simulink model "global_model"  (R2021a)
settings: Solver=ode8  StartTime=0.0  StopTime=205  FixedStep=0.1  RelTol=1e-3  EnableMultiTasking=on
undefined symbols (not defined in the file or in its folder): sigbuilder_block
settings Model: Creator=Lu  LastModifiedBy=10365
settings SolverCC: ZeroCrossAlgorithm=Adaptive  AlgebraicLoopSolver=TrustRegion
settings DataIOCC: LimitDataPoints=on  MaxDataPoints=10000  SaveFormat=Array  ReturnWorkspaceOutputs=off
settings OptimizationCC: ExpressionDepthLimit=2147483647  LifeSpan=inf
settings DebuggingCC: UnderspecifiedInitializationDetection=Classic  MergeDetectMultiDrivingBlocksExec=none  SolverPrmCheckMsg=warning  StateNameClashWarn=warning  SFUnexpectedBacktrackingDiag=warning  SFNoUnconditionalDefaultTransitionDiag=warning  SFExecutionAtInitializationDiag=none  SFMachineParentedDataDiag=warning  ArithmeticOperatorsInVariantConditions=warning
settings HardwareCC: ProdBitPerPointer=32  ProdBitPerSizeT=32  ProdBitPerPtrDiffT=32  ProdLargestAtomicFloat=None  ProdIntDivRoundTo=Undefined  ProdEndianess=Unspecified  ProdWordSize=32  ProdHWDeviceType=32-bit Generic
settings ModelReferenceCC: PropagateSignalLabelsOutOfModel=off
settings SFSimCC: SimUseLocalCustomCode=off  CustomCodeUndefinedFunction=UseInterfaceOnly
settings RTWCC: RTWUseLocalCustomCode=off
settings CodeAppCC: StateflowObjectComments=on
settings GRTTargetCC: TargetLangStandard=C89/C90 (ANSI)
settings ConfigComp: CovMetricSettings=dw  CovSaveCumulativeToWorkspaceVar=on  CovSaveSingleToWorkspaceVar=on  CovExternalEMLEnable=off

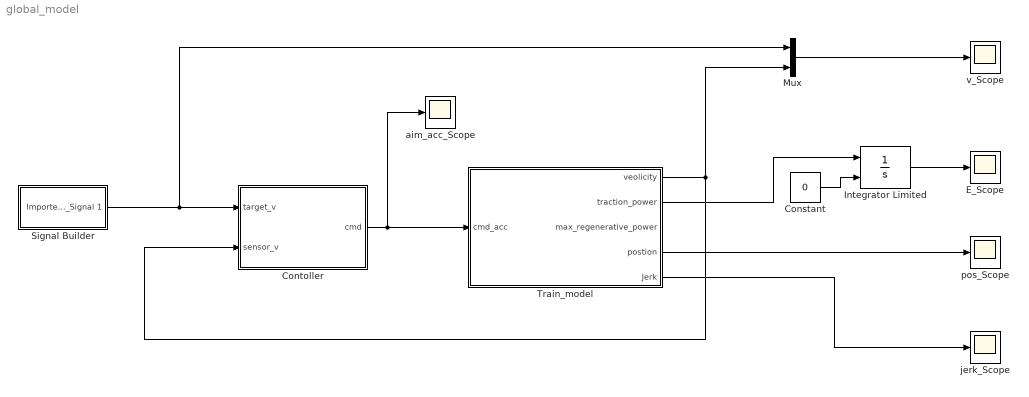
== system global_model ==
  Constant : Constant  Value=0
  Contoller : Subsystem
  E_Scope : Scope
  Integrator Limited : Integrator  InitialConditionSource=external  LimitOutput=on  LowerSaturationLimit=0
  Mux : Mux  Inputs=2
  Signal Builder : Subsystem  Tag=STV Subsys  LoadFcn=sigbuilder_block('load');  StartFcn=sigbuilder_block('start');  StopFcn=sigbuilder_block('stop');  ClipboardFcn=sigbuilder_block('clipboard');  mask(Sigbuilder block){tuvar=[0:10]}
      mask help: Simulink:masks:SigbuilderBlock_MD
      mask init:
      | if ~strcmp(get_param(bdroot(gcbh),'SimulationStatus'),'stopped') tuvar = sigbuilder_block('maskInit'); end
      settings: CopyFcn=sigbuilder_block('copy');  DeleteFcn=sigbuilder_block('delete');  ModelCloseFcn=sigbuilder_block('modelClose');  PreSaveFcn=sigbuilder_block('preSave');  PauseFcn=sigbuilder_block('pause');  ContinueFcn=sigbuilder_block('continue');  NameChangeFcn=sigbuilder_block('namechange');  OpenFcn=sigbuilder_block('open',[437.6 186.6 575.8 400.2 ]);  CloseFcn=sigbuilder_block('close');
      mask Display: plot(0, 0, 100, 100,[2, 2, 32, 32, 2], [68, 8, 8, 68, 68],[32, 2], [38, 38], [32, 19, 2],[53, 60, 44], [32, 17, 17, 2],[16, 16, 31, 31]);txt = getActiveGroup(gcbh);text(2, 100, txt,'verticalAlignment', 'top');
  Train_model : Subsystem
  aim_acc_Scope : Scope
  jerk_Scope : Scope
  pos_Scope : Scope
  v_Scope : Scope
  wires:
  Contoller/1(cmd) -> aim_acc_Scope/1, Train_model/1(cmd_acc)
  Train_model/1(veolicity) -> Contoller/2(sensor_v), Mux/2
  Signal Builder/1(Imported_Signal 1) -> Mux/1, Contoller/1(target_v)
  Integrator Limited/1 -> E_Scope/1
  Train_model/2(traction_power) -> Integrator Limited/1
  Train_model/4(postion) -> pos_Scope/1
  Mux/1 -> v_Scope/1
  Constant/1 -> Integrator Limited/2
  Train_model/5(Jerk) -> jerk_Scope/1

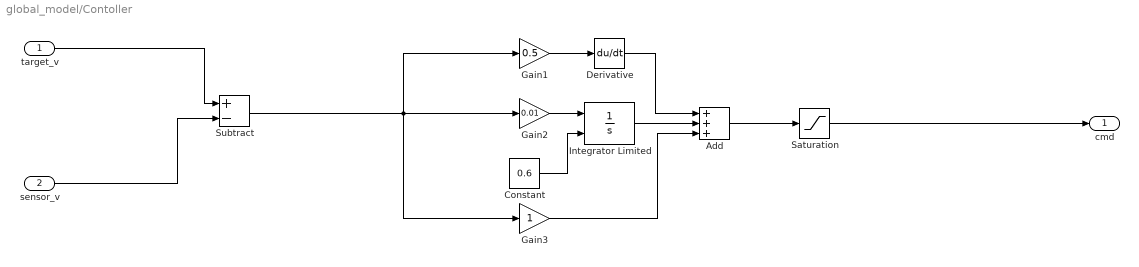
== system global_model/Contoller ==
  target_v : Inport
  sensor_v : Inport  Port=2
  Add : Sum  Inputs=+++
  Constant : Constant  Value=0.6
  Derivative : Derivative
  Gain1 : Gain  Gain=0.5
  Gain2 : Gain  Gain=0.01
  Gain3 : Gain
  Integrator Limited : Integrator  InitialConditionSource=external  LimitOutput=on  LowerSaturationLimit=0
  Saturation : Saturate  UpperLimit=1  LowerLimit=-1
  Subtract : Sum  Inputs=+-
  cmd : Outport  VectorParamsAs1DForOutWhenUnconnected=off
  wires:
  sensor_v/1 -> Subtract/2
  Gain2/1 -> Integrator Limited/1
  Subtract/1 -> Gain1/1, Gain3/1, Gain2/1
  Gain1/1 -> Derivative/1
  Integrator Limited/1 -> Add/2
  Derivative/1 -> Add/1
  Gain3/1 -> Add/3
  Add/1 -> Saturation/1
  target_v/1 -> Subtract/1
  Saturation/1 -> cmd/1
  Constant/1 -> Integrator Limited/2

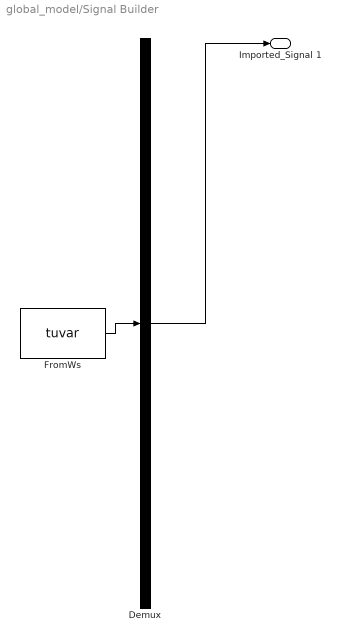
== system global_model/Signal Builder ==
  Demux : Demux  Tag=STV Demux  Outputs=1
      settings: DisplayOption=none
  FromWs : FromWorkspace  Tag=STV FromWs  VariableName=tuvar
      SigBuilderData=|
      | common.afterFinalStr = 'Extrapolate'
      | common.sampleTime = 0
      | dataSet.timeRange = [0 205]
      | dataSet.name = 'Sheet1'
      | sbobj.Groups.Name = 'Sheet1'
      | sbobj.Groups.Signals.Name = 'Imported_Signal 1'
      | sbobj.Groups.Signals.XData = [0 0.5 1 1.5 2 2.5 3 3.5 4 4.5 5 5.5 6 6.5 7 7.5 8 8.5 9 9.5 10 10.5 11 11.5 12 12.5 13 13.5 14 14.5 15 15.5 16 16.5 17 17.5 18 18.5 19 19.5 20 20.5 21 21.5 22 22.5 23 23.5 24 24.5 25 25.5 26 26.5 27 27.5 28 28.5 29 29.5 30 30.5 31 31.5 32 32.5 33 33.5 34 34.5 35 35.5 36 36.5 37 37.5 38 38.5 39 39.5 40 40.5 41 41.5 42 42.5 43 43.5 44 44.5 45 45.5 46 46.5 47 47.5 48 48.5 49 49.5 50 50.5 51 51.5 52 52.5 53 53.5 54 54.5 55 55.5 56 56.5 57 57.5 58 58.5 59 59.5 60 60.5 61 61.5 62 62.5 63 63.5 64 64.5 65 65.5 66 66.5 67 67.5 68 68.5 69 69.5 70 70.5 71 71.5 72 72.5 73 73.5 74 74.5 75 75.5 76 76.5 77 77.5 78 78.5 79 79.5 80 80.5 81 81.5 82 82.5 83 83.5 84 84.5 85 85.5 86 86.5 87 87.5 88 88.5 89 89.5 90 90.5 91 91.5 92 92.5 93 93.5 94 94.5 95 95.5 96 96.5 97 97.5 98 98.5 99 99.5 100 100.5 101 101.5 102 102.5 103 103.5 104 104.5 105 105.5 106 106.5 107 107.5 108 108.5 109 109.5 110 110.5 111 111.5 112 112.5 113 113.5 114 114.5 115 115.5 116 116.5 117 117.5 118 118.5 119 119.5 120 120.5 121 121.5 122 122.5 123 123.5 124 124.5 125 125.5 126 126.5 127 127.5 128 128.5 129 129.5 130 130.5 131 131.5 132 132.5 133 133.5 134 134.5 135 135.5 136 136.5 137 137.5 138 138.5 139 139.5 140 140.5 141 141.5 142 142.5 143 143.5 144 144.5 145 145.5 146 146.5 147 147.5 148 148.5 149 149.5 150 150.5 151 151.5 152 152.5 153 153.5 154 154.5 155 155.5 156 156.5 157 157.5 158 158.5 159 159.5 160 160.5 161 161.5 162 162.5 163 163.5 164 164.5 165 165.5 166 166.5 167 167.5 168 168.5 169 169.5 170 170.5 171 171.5 172 172.5 173 173.5 174 174.5 175 175.5 176 176.5 177 177.5 178 178.5 179 179.5 180 180.5 181 181.5 182 182.5 183 183.5 184 185 185.5 186 186.5 187 187.5 188 188.5 189 189.5 190 190.5 191 191.5 192 192.5 193 193.5 194 195 195.5 196 196.5 197 197.5 198 198.5 199 199.5 200 200.5 201 201.5 202 202.5 203 203.5 204 204.5 205]
      | sbobj.Groups.Signals.YData = [0 0.25 0.625 1.125 1.6460007206 2.16641322842 2.6862319684 3.20545141303 3.7240660625 4.24207044493 4.75945911658 5.27622666204 ... (409 elements, 1x409)]
      | sbobj.Groups.TimeRange = [0 205]
  Imported_Signal 1 : Outport  Tag=STV Outport  VectorParamsAs1DForOutWhenUnconnected=off
  wires:
  Demux/1 -> Imported_Signal 1/1
  FromWs/1 -> Demux/1

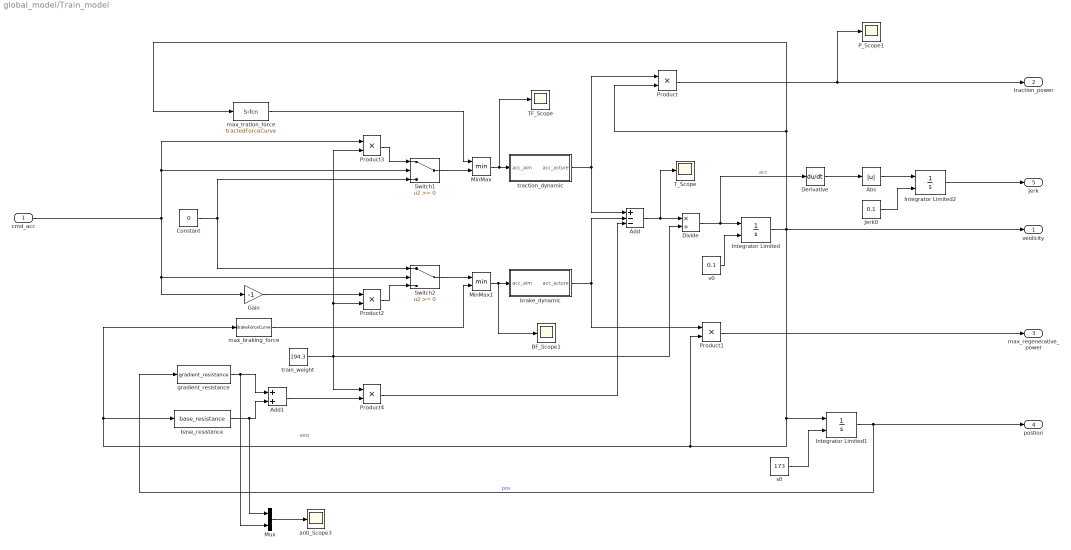
== system global_model/Train_model ==
  note: veo
  cmd_acc : Inport
  Abs : Abs
  Add : Sum  Inputs=+--
  Add1 : Sum
  BF_Scope1 : Scope
  Constant : Constant  Value=0
  Derivative : Derivative  CoefficientInTFapproximation=100
  Divide : Product  Inputs=*/
  Gain : Gain  Gain=-1
  Integrator Limited : Integrator  InitialConditionSource=external  LimitOutput=on  LowerSaturationLimit=0
  Integrator Limited1 : Integrator  InitialConditionSource=external  LimitOutput=on  LowerSaturationLimit=0
  Integrator Limited2 : Integrator  InitialConditionSource=external  LimitOutput=on  LowerSaturationLimit=0
  Jerk0 : Constant  Value=0.1
  MinMax : MinMax  Inputs=2
  MinMax1 : MinMax  Inputs=2
  Mux : Mux  Inputs=2
  P_Scope1 : Scope
  Product{,1..4} (5 alike) : Product
  Switch1 : Switch
  Switch2 : Switch
  TF_Scope : Scope
  T_Scope : Scope
  anti_Scope3 : Scope
  base_resistance : S-Function  FunctionName=base_resistance  SFunctionDeploymentMode=off  EnableBusSupport=off
  brake_dynamic : Subsystem
  gradient_resistance : S-Function  FunctionName=gradient_resistance  SFunctionDeploymentMode=off  EnableBusSupport=off
  max_braking_force : S-Function  FunctionName=BrakeForceCurve  SFunctionDeploymentMode=off  EnableBusSupport=off
  max_tration_force : S-Function  FunctionName=tractedForceCurve  SFunctionDeploymentMode=off  EnableBusSupport=off
  s0 : Constant  Value=173
  traction_dynamic : Subsystem
  train_weight : Constant  Value=194.3
  v0 : Constant  Value=0.1
  veolicity : Outport  VectorParamsAs1DForOutWhenUnconnected=off
  traction_power : Outport  Port=2  VectorParamsAs1DForOutWhenUnconnected=off
  max_regenerative_power : Outport  Port=3  VectorParamsAs1DForOutWhenUnconnected=off
  postion : Outport  Port=4  VectorParamsAs1DForOutWhenUnconnected=off
  Jerk : Outport  Port=5  VectorParamsAs1DForOutWhenUnconnected=off
  wires:
  v0/1 -> Integrator Limited/2
  Constant/1 -> Switch2/1, Switch1/3
  brake_dynamic/1(acc_acture) -> Product1/1, Add/2
  traction_dynamic/1(acc_acture) -> Product/1, Add/1
  MinMax/1 -> TF_Scope/1, traction_dynamic/1(acc_aim)
  Switch1/1 -> MinMax/2
  Switch2/1 -> MinMax1/1
  max_tration_force/1 -> MinMax/1
  Integrator Limited1/1 -> postion/1, gradient_resistance/1  "pos"
  gradient_resistance/1 -> Mux/2, Add1/1
  base_resistance/1 -> Mux/1, Add1/2
  max_braking_force/1 -> MinMax1/2
  Product/1 -> P_Scope1/1, traction_power/1
  Integrator Limited/1 -> Integrator Limited1/1, base_resistance/1, max_braking_force/1, Product1/2, Product/2, max_tration_force/1, veolicity/1
  Divide/1 -> Derivative/1, Integrator Limited/1  "acc"
  train_weight/1 -> Product4/1, Product3/2, Product2/2, Divide/2
  Product1/1 -> max_regenerative_power/1
  Product2/1 -> Switch2/3
  Product3/1 -> Switch1/1
  cmd_acc/1 -> Gain/1, Switch2/2, Product3/1, Switch1/2
  Add1/1 -> Product4/2
  Product4/1 -> Add/3
  s0/1 -> Integrator Limited1/2
  Add/1 -> T_Scope/1, Divide/1
  Gain/1 -> Product2/1
  MinMax1/1 -> BF_Scope1/1, brake_dynamic/1(acc_aim)
  Abs/1 -> Integrator Limited2/1
  Jerk0/1 -> Integrator Limited2/2
  Integrator Limited2/1 -> Jerk/1
  Derivative/1 -> Abs/1
  Mux/1 -> anti_Scope3/1

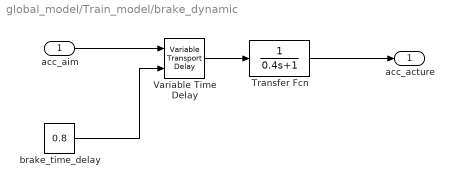
== system global_model/Train_model/brake_dynamic ==
  acc_aim : Inport
  Transfer Fcn : TransferFcn  Denominator=[0.4 1]
  Variable Time Delay : VariableTransportDelay  MaximumDelay=10
  brake_time_delay : Constant  Value=0.8
  acc_acture : Outport  VectorParamsAs1DForOutWhenUnconnected=off
  wires:
  Variable Time Delay/1 -> Transfer Fcn/1
  acc_aim/1 -> Variable Time Delay/1
  Transfer Fcn/1 -> acc_acture/1
  brake_time_delay/1 -> Variable Time Delay/2

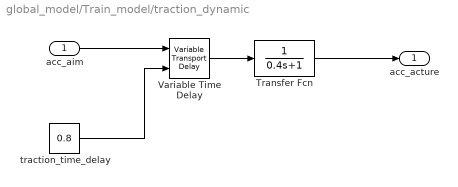
== system global_model/Train_model/traction_dynamic ==
  acc_aim : Inport
  Transfer Fcn : TransferFcn  Denominator=[0.4 1]
  Variable Time Delay : VariableTransportDelay  MaximumDelay=10
  traction_time_delay : Constant  Value=0.8
  acc_acture : Outport  VectorParamsAs1DForOutWhenUnconnected=off
  wires:
  acc_aim/1 -> Variable Time Delay/1
  Variable Time Delay/1 -> Transfer Fcn/1
  Transfer Fcn/1 -> acc_acture/1
  traction_time_delay/1 -> Variable Time Delay/2
